simulink subsystem "PvtSubSys_VSM_LCKIE"  (R2020b)
settings: Solver=VariableStepAuto  StartTime=0.0  StopTime=10.0  RelTol=1e-3
values from neighbouring files (symbols this model uses):
  P_VSM_LCKIE_ClassInput = 0.0    [LCKIE.sldd]
  P_VSM_LCKIE_Laneoffset : value not decoded    [LCKIE.sldd]
  P_VSM_LCKIE_Laneoffset_BP : value not decoded    [LCKIE.sldd]
  P_VSM_LCKIE_LatC_DisOffofLanWidth : value not decoded    [LCKIE.sldd]
  P_VSM_LCKIE_LatC_DisOffofSpd : value not decoded    [LCKIE.sldd]
  P_VSM_LCKIE_LatC_DisSW = 0.0    [LCKIE.sldd]
  P_VSM_LCKIE_LatC_LanWidth : value not decoded    [LCKIE.sldd]
  P_VSM_LCKIE_LATC_LimitDis : value not decoded    [LCKIE.sldd]
  P_VSM_LCKIE_LATC_LimitDis_BP : value not decoded    [LCKIE.sldd]
  P_VSM_LCKIE_LatC_LimitDisEgoToObjSelt = 1.5    [LCKIE.sldd]
  P_VSM_LCKIE_LatC_LimitEgoToOppLane = 0.3    [LCKIE.sldd]
  P_VSM_LCKIE_LatC_maxLimitDisREToLane = 2.5    [LCKIE.sldd]
  P_VSM_LCKIE_LatC_minLimitDisREToLane = 1.2    [LCKIE.sldd]
  P_VSM_LCKIE_LatC_MoveEnableDis = 0.0    [LCKIE.sldd]
  P_VSM_LCKIE_LatC_RESafDis = 0.8    [LCKIE.sldd]
  P_VSM_LCKIE_LatC_SafeDisofLanWidth : value not decoded    [LCKIE.sldd]
  P_VSM_LCKIE_LatC_Spd : value not decoded    [LCKIE.sldd]
  P_VSM_LCKIE_LongC_d1 : value not decoded    [LCKIE.sldd]
  P_VSM_LCKIE_LongC_d2 : value not decoded    [LCKIE.sldd]
  P_VSM_LCKIE_LongC_DetaSpd : value not decoded    [LCKIE.sldd]
  P_VSM_LCKIE_LongC_DirecChangeDis = 20.0    [LCKIE.sldd]
  P_VSM_LCKIE_LongC_FleetOff = 80.0    [LCKIE.sldd]
  P_VSM_LCKIE_LongC_maxDis = 80.0    [LCKIE.sldd]
  P_VSM_LCKIE_LongC_minDis = 50.0    [LCKIE.sldd]
  P_VSM_LCKIE_LongC_ShutDownLongDis = -25.0    [LCKIE.sldd]
  P_VSM_LCKIE_LongC_ShutDownTTC = -4.0    [LCKIE.sldd]
  P_VSM_LCKIE_LongC_Spd : value not decoded    [LCKIE.sldd]
  P_VSM_LCKIE_LongC_toff = 10.0    [LCKIE.sldd]
  P_VSM_LCKIE_OFC_ActDis = 10.0    [LCKIE.sldd]
  P_VSM_LCKIE_OFC_DownDis = 10.0    [LCKIE.sldd]
  P_VSM_LCKIE_OFC_DownTTC = 5.0    [LCKIE.sldd]
  P_VSM_LCKIE_OFC_SafDis = 10.0    [LCKIE.sldd]
  P_VSM_LCKIE_OFC_Toff = 3.0    [LCKIE.sldd]
  P_VSM_LCKIE_ORC_LatDis = 1.8    [LCKIE.sldd]
  P_VSM_LCKIE_ORC_LimitDis1 = -30.0    [LCKIE.sldd]
  P_VSM_LCKIE_ORC_LimitDis2 = -10.0    [LCKIE.sldd]
  P_VSM_LCKIE_ORC_LimitTTC = 10.0    [LCKIE.sldd]
  P_VSM_LCKIE_ORC_LowSpd = -5.0    [LCKIE.sldd]
  P_VSM_LCKIE_POC_Delaytime : value not decoded    [LCKIE.sldd]
  P_VSM_LCKIE_POC_detaSpd : value not decoded    [LCKIE.sldd]
  P_VSM_LCKIE_POC_LimitDis = -15.0    [LCKIE.sldd]
  P_VSM_LCKIE_POC_LimitTTC = 2.0    [LCKIE.sldd]
  P_VSM_LCKIE_State_CurveMax = 0.005    [LCKIE.sldd]
  P_VSM_LCKIE_State_CurveMin = 0.0055555555555555558    [LCKIE.sldd]
  P_VSM_LCKIE_State_detaspd = 1.39    [LCKIE.sldd]
  P_VSM_LCKIE_State_detaspd_enable = 1.0    [LCKIE.sldd]
  P_VSM_LCKIE_State_DriverInputTrqValue_enable = 1.0    [LCKIE.sldd]
  P_VSM_LCKIE_State_ELKObjClc = 1.0    [LCKIE.sldd]
  P_VSM_LCKIE_State_HWASts_disable = 1.0    [LCKIE.sldd]
  P_VSM_LCKIE_State_IEObjClc = 1.0    [LCKIE.sldd]
  P_VSM_LCKIE_State_IFVReady = 1.0    [LCKIE.sldd]
  P_VSM_LCKIE_State_lamb_enable = 1.0    [LCKIE.sldd]
  P_VSM_LCKIE_State_Lanecurve_enable = 1.0    [LCKIE.sldd]
  P_VSM_LCKIE_State_LaneWidth_enable = 1.0    [LCKIE.sldd]
  P_VSM_LCKIE_State_Off2on = 3.0    [LCKIE.sldd]
  P_VSM_LCKIE_State_OppObjClc = 1.0    [LCKIE.sldd]
  P_VSM_LCKIE_STATE_ORCObjenable = 0.0    [LCKIE.sldd]
  P_VSM_LCKIE_State_Vehspeed_enable = 1.0    [LCKIE.sldd]
  P_VSM_LCKIE_State_wiper_enable = 1.0    [LCKIE.sldd]
  P_VSM_LCKIE_tcycle = 0.02    [LCKIE.sldd]
undefined symbols (not defined in the file or in its folder): P_Global_Vehicle_Length_m, P_Global_VehicleWidthMin_m, P_VSM_LSMC_SampleTime, STATE
libraries: simulink x62
(part 1 of 5)
settings Model: Creator=GW00133806  LastModifiedBy=GW00201118

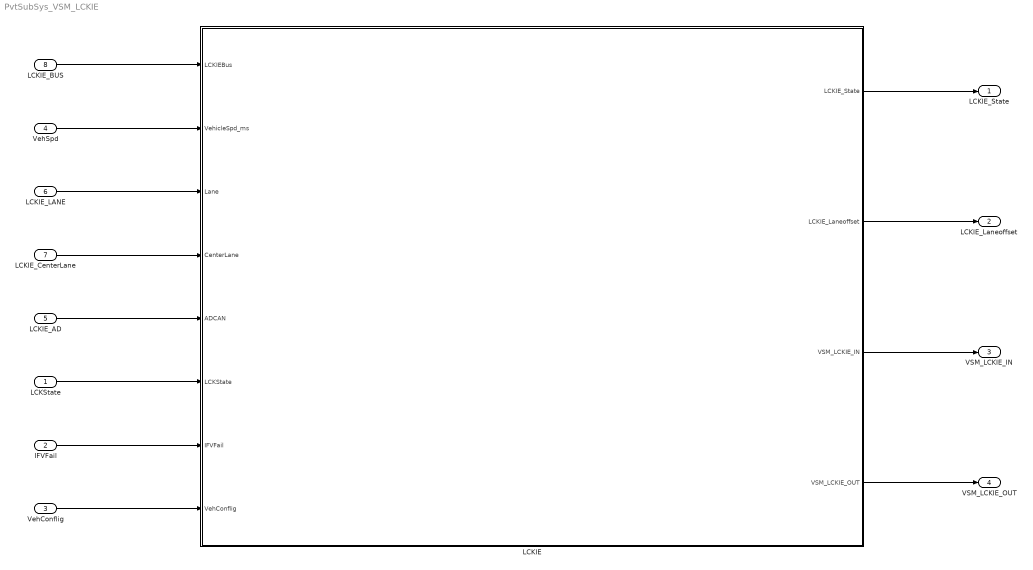
== system PvtSubSys_VSM_LCKIE ==
  LCKState : Inport
  IFVFail : Inport  Port=2
  VehConflig : Inport  Port=3
  VehSpd : Inport  Port=4
  LCKIE_AD : Inport  Port=5  OutDataTypeStr=Bus: LCKIE_AD  BusOutputAsStruct=on
  LCKIE_LANE : Inport  Port=6  BusOutputAsStruct=on
  LCKIE_CenterLane : Inport  Port=7  OutDataTypeStr=Bus: CenterLane  BusOutputAsStruct=on
  LCKIE_BUS : Inport  Port=8  OutDataTypeStr=Bus: TOS_LCKIE_BUS  BusOutputAsStruct=on
  LCKIE : Subsystem
  LCKIE_State : Outport
  LCKIE_Laneoffset : Outport  Port=2
  VSM_LCKIE_IN : Outport  Port=3
  VSM_LCKIE_OUT : Outport  Port=4
  wires:
  LCKIE/2(LCKIE_Laneoffset) -> LCKIE_Laneoffset/1
  LCKState/1 -> LCKIE/6(LCKState)
  LCKIE/3(VSM_LCKIE_IN) -> VSM_LCKIE_IN/1
  LCKIE_CenterLane/1 -> LCKIE/4(CenterLane)
  VehConflig/1 -> LCKIE/8(VehConflig)
  LCKIE/1(LCKIE_State) -> LCKIE_State/1
  LCKIE_BUS/1 -> LCKIE/1(LCKIEBus)
  VehSpd/1 -> LCKIE/2(VehicleSpd_ms)
  IFVFail/1 -> LCKIE/7(IFVFail)
  LCKIE/4(VSM_LCKIE_OUT) -> VSM_LCKIE_OUT/1
  LCKIE_LANE/1 -> LCKIE/3(Lane)
  LCKIE_AD/1 -> LCKIE/5(ADCAN)

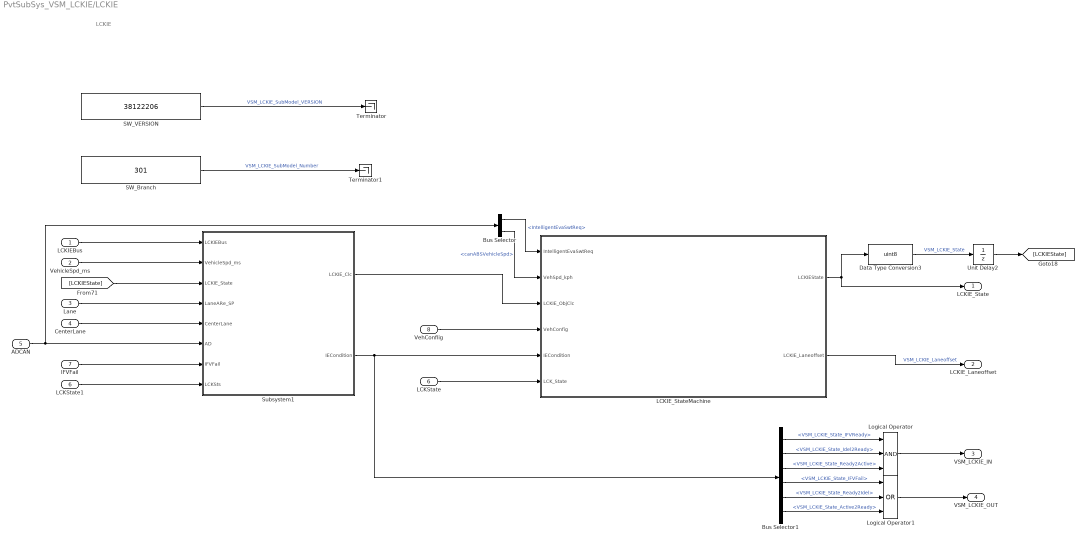
== system PvtSubSys_VSM_LCKIE/LCKIE ==
  note: LCKIE
  LCKIEBus : Inport
  VehicleSpd_ms : Inport  Port=2
  Lane : Inport  Port=3
  CenterLane : Inport  Port=4
  ADCAN : Inport  Port=5
  LCKState : Inport  Port=6
  IFVFail : Inport  Port=7
  VehConflig : Inport  Port=8
  Bus Selector : BusSelector  OutputSignals=IntelligentEvaSwtReq,canABSVehicleSpd
  Bus Selector1 : BusSelector  OutputSignals=VSM_LCKIE_State_IFVReady,VSM_LCKIE_State_Idel2Ready,VSM_LCKIE_State_Ready2Active,VSM_LCKIE_State_IFVFail,VSM_LCKIE_State_Ready2Idel,VSM_LCKIE_State_Active2Ready
  Data Type Conversion3 : DataTypeConversion  OutDataTypeStr=uint8
  LCKIE_StateMachine : Subsystem
  LCKState1 : InportShadow  Port=6
  Logical Operator : Logic  Inputs=3  AllPortsSameDT=off  OutDataTypeStr=boolean
  Logical Operator1 : Logic  Operator=OR  Inputs=3  AllPortsSameDT=off  OutDataTypeStr=boolean
  SW_Branch : Constant  Value=301  OutDataTypeStr=uint16
  SW_VERSION : Constant  Value=38122206  OutDataTypeStr=uint32
  Subsystem1 : Subsystem
  Terminator : Terminator
  Terminator1 : Terminator
  Unit Delay2 : UnitDelay  SampleTime=-1  HasFrameUpgradeWarning=on
  LCKIE_State : Outport
  LCKIE_Laneoffset : Outport  Port=2
  VSM_LCKIE_IN : Outport  Port=3
  VSM_LCKIE_OUT : Outport  Port=4
  wires:
  SW_Branch/1 -> Terminator1/1  "VSM_LCKIE_SubModel_Number"
  Bus Selector/1 -> LCKIE_StateMachine/1(IntelligentEvaSwtReq)  "<IntelligentEvaSwtReq>"
  Logical Operator1/1 -> VSM_LCKIE_OUT/1
  Logical Operator/1 -> VSM_LCKIE_IN/1
  Bus Selector1/6 -> Logical Operator1/3  "<VSM_LCKIE_State_Active2Ready>"
  Bus Selector1/5 -> Logical Operator1/2  "<VSM_LCKIE_State_Ready2Idel>"
  Bus Selector1/4 -> Logical Operator1/1  "<VSM_LCKIE_State_IFVFail>"
  Bus Selector1/3 -> Logical Operator/3  "<VSM_LCKIE_State_Ready2Active>"
  Bus Selector1/2 -> Logical Operator/2  "<VSM_LCKIE_State_Idel2Ready>"
  Bus Selector1/1 -> Logical Operator/1  "<VSM_LCKIE_State_IFVReady>"
  VehConflig/1 -> LCKIE_StateMachine/4(VehConfig)
  CenterLane/1 -> Subsystem1/5(CenterLane)
  Lane/1 -> Subsystem1/4(LaneARe_SP)
  VehicleSpd_ms/1 -> Subsystem1/2(VehicleSpd_ms)
  IFVFail/1 -> Subsystem1/7(IFVFail)
  Unit Delay2/1 -> [LCKIEState]
  ADCAN/1 -> Subsystem1/6(AD), Bus Selector/1
  LCKIE_StateMachine/1(LCKIEState) -> Data Type Conversion3/1, LCKIE_State/1
  Subsystem1/2(IECondition) -> Bus Selector1/1, LCKIE_StateMachine/5(IECondition)
  Subsystem1/1(LCKIE_Clc) -> LCKIE_StateMachine/3(LCKIE_ObjClc)
  Data Type Conversion3/1 -> Unit Delay2/1  "VSM_LCKIE_State"
  [LCKIEState] -> Subsystem1/3(LCKIE_State)
  LCKState/1 -> LCKIE_StateMachine/6(LCK_State)
  LCKIEBus/1 -> Subsystem1/1(LCKIEBus)
  LCKIE_StateMachine/2(LCKIE_Laneoffset) -> LCKIE_Laneoffset/1  "VSM_LCKIE_Laneoffset"
  SW_VERSION/1 -> Terminator/1  "VSM_LCKIE_SubModel_VERSION"
  LCKState1/1 -> Subsystem1/8(LCKSts)
  Bus Selector/2 -> LCKIE_StateMachine/2(VehSpd_kph)  "<canABSVehicleSpd>"

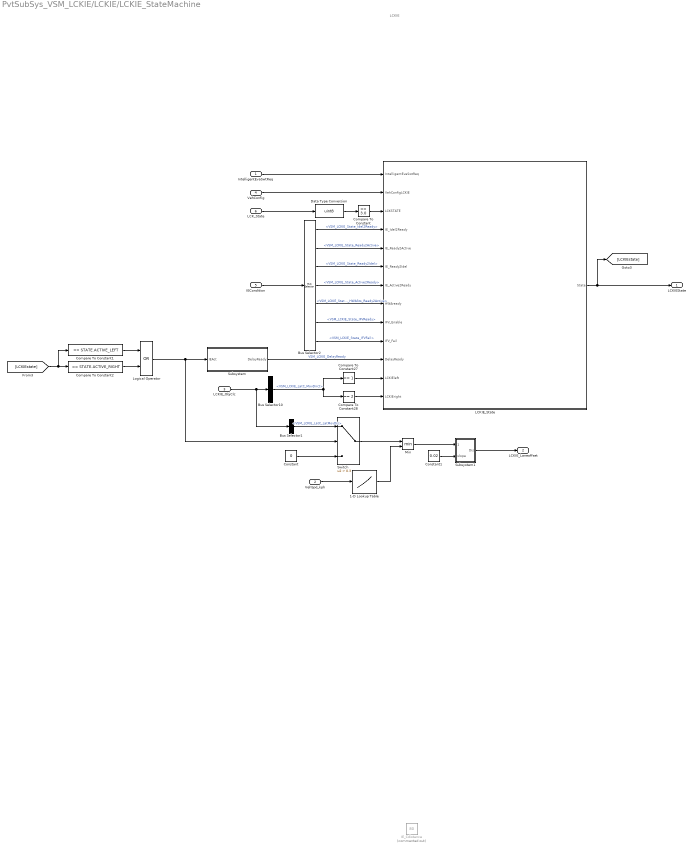
== system PvtSubSys_VSM_LCKIE/LCKIE/LCKIE_StateMachine ==
  note: LCKIE
  IntelligentEvaSwtReq : Inport
  VehSpd_kph : Inport  Port=2
  LCKIE_ObjClc : Inport  Port=3
  VehConfig : Inport  Port=4
  IECondition : Inport  Port=5
  LCK_State : Inport  Port=6
  1-D Lookup Table : Lookup_n-D  NumberOfTableDimensions=1  BreakpointsForDimension1=P_VSM_LCKIE_Laneoffset_BP  Table=P_VSM_LCKIE_Laneoffset  ExtrapMethod=Clip  UseLastTableValue=on  InternalRulePriority=Speed  RndMeth=Simplest  InputSameDT=on
  Bus Selector1 : BusSelector  OutputSignals=VSM_LCKIE_LatC_LatMovDis
  Bus Selector10 : BusSelector  OutputSignals=VSM_LCKIE_LatC_MovDirct
  Bus Selector2 : BusSelector  OutputSignals=VSM_LCKIE_State_Idel2Ready,VSM_LCKIE_State_Ready2Active,VSM_LCKIE_State_Ready2Idel,VSM_LCKIE_State_Active2Ready,VSM_LCKIE_State_HWASts_Ready2Active,VSM_LCKIE_State_IFVReady,VSM_LCKIE_State_IFVFail
  Compare To Constant : simulink/Logic and Bit Operations/Compare To Constant  relop===  const=3.0  OutDataTypeStr=boolean
  Compare To Constant1 : simulink/Logic and Bit Operations/Compare To Constant  relop===  const=STATE.ACTIVE_LEFT  OutDataTypeStr=boolean
  Compare To Constant2 : simulink/Logic and Bit Operations/Compare To Constant  relop===  const=STATE.ACTIVE_RIGHT  OutDataTypeStr=boolean
  Compare To Constant27 : simulink/Logic and Bit Operations/Compare To Constant  relop===  const=1  OutDataTypeStr=boolean
  Compare To Constant28 : simulink/Logic and Bit Operations/Compare To Constant  relop===  const=2  OutDataTypeStr=boolean
  Constant : Constant  Value=0
  Constant1 : Constant  Value=0.02  OutDataTypeStr=single
  Data Type Conversion : DataTypeConversion  OutDataTypeStr=uint8
  IE_Cdistance : Constant  Commented=on  Value=80
  LCKIE_State : Stateflow chart  TreatAsAtomicUnit=on
  Logical Operator : Logic  Operator=OR  AllPortsSameDT=off  OutDataTypeStr=boolean
  Min : MinMax  Inputs=2
  Subsystem : Subsystem
  Subsystem1 : Subsystem
  Switch : Switch  Criteria=u2 > Threshold  Threshold=0.3  OutDataTypeStr=single
  LCKIEState : Outport
  LCKIE_Laneoffset : Outport  Port=2
  wires:
  Compare To Constant/1 -> LCKIE_State/3(LCKSTATE)
  Switch/1 -> Min/1
  LCKIE_State/1(State) -> [LCKIEstate], LCKIEState/1
  Compare To Constant1/1 -> Logical Operator/1
  Compare To Constant2/1 -> Logical Operator/2
  Constant/1 -> Switch/3
  Compare To Constant28/1 -> LCKIE_State/13(LCKIEright)
  IntelligentEvaSwtReq/1 -> LCKIE_State/1(IntelligentEvaSwtReq)
  LCK_State/1 -> Data Type Conversion/1
  Compare To Constant27/1 -> LCKIE_State/12(LCKIEleft)
  Bus Selector10/1 -> Compare To Constant28/1, Compare To Constant27/1  "<VSM_LCKIE_LatC_MovDirct>"
  Data Type Conversion/1 -> Compare To Constant/1
  [LCKIEstate] -> Compare To Constant2/1, Compare To Constant1/1
  VehConfig/1 -> LCKIE_State/2(VehConfigLCKIE)
  Min/1 -> Subsystem1/1(DisLimmit)
  Bus Selector1/1 -> Switch/1  "<VSM_LCKIE_LatC_LatMovDis>"
  IECondition/1 -> Bus Selector2/1
  Bus Selector2/2 -> LCKIE_State/5(IE_Ready2Active)  "<VSM_LCKIE_State_Ready2Active>"
  Bus Selector2/1 -> LCKIE_State/4(IE_Idel2Ready)  "<VSM_LCKIE_State_Idel2Ready>"
  Bus Selector2/3 -> LCKIE_State/6(IE_Ready2Idel)  "<VSM_LCKIE_State_Ready2Idel>"
  Bus Selector2/4 -> LCKIE_State/7(IE_Active2Ready)  "<VSM_LCKIE_State_Active2Ready>"
  Bus Selector2/6 -> LCKIE_State/9(IFV_Enable)  "<VSM_LCKIE_State_IFVReady>"
  Bus Selector2/7 -> LCKIE_State/10(IFV_Fail)  "<VSM_LCKIE_State_IFVFail>"
  Subsystem1/1(Dis) -> LCKIE_Laneoffset/1
  Constant1/1 -> Subsystem1/2(slope)
  Bus Selector2/5 -> LCKIE_State/8(HWAready)  "<VSM_LCKIE_State_HWASts_Ready2Active>"
  Logical Operator/1 -> Switch/2, Subsystem/1(IEAct)
  Subsystem/1(DelayReady) -> LCKIE_State/11(DelayReady)  "VSM_LCKIE_DelayReady"
  LCKIE_ObjClc/1 -> Bus Selector1/1, Bus Selector10/1
  VehSpd_kph/1 -> 1-D Lookup Table/1
  1-D Lookup Table/1 -> Min/2

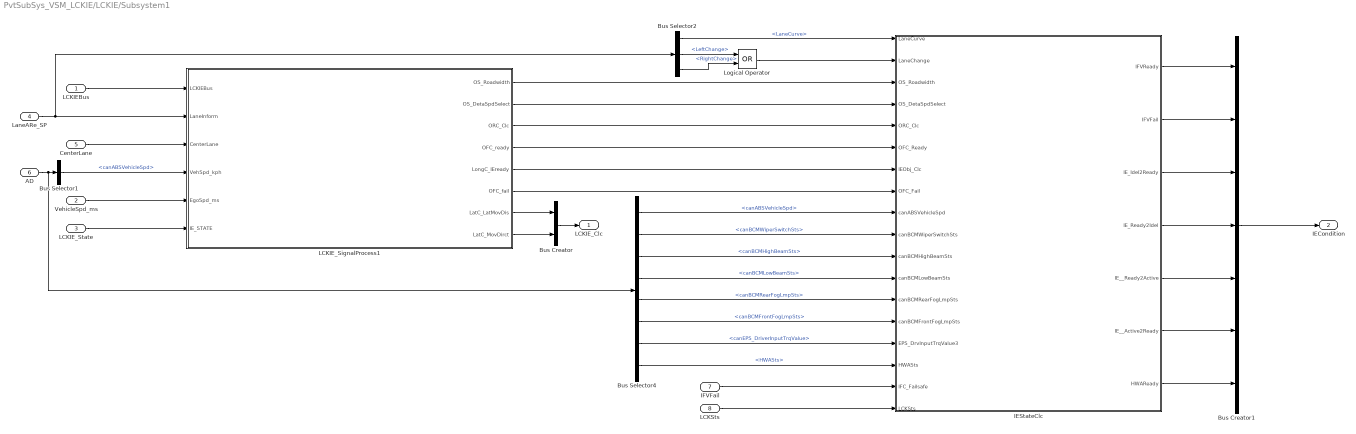
== system PvtSubSys_VSM_LCKIE/LCKIE/Subsystem1 ==
  LCKIEBus : Inport
  VehicleSpd_ms : Inport  Port=2
  LCKIE_State : Inport  Port=3
  LaneARe_SP : Inport  Port=4
  CenterLane : Inport  Port=5
  AD : Inport  Port=6
  IFVFail : Inport  Port=7
  LCKSts : Inport  Port=8
  Bus Creator : BusCreator  Inputs=2
  Bus Creator1 : BusCreator  Inputs=7
  Bus Selector1 : BusSelector  OutputSignals=canABSVehicleSpd
  Bus Selector2 : BusSelector  OutputSignals=LaneCurve,LeftChange,RightChange
  Bus Selector4 : BusSelector  OutputSignals=canABSVehicleSpd,canBCMWiperSwitchSts,canBCMHighBeamSts,canBCMLowBeamSts,canBCMRearFogLmpSts,canBCMFrontFogLmpSts,canEPS_DriverInputTrqValue,HWASts
  IEStateClc : Subsystem
  LCKIE_SignalProcess1 : Subsystem
  Logical Operator : Logic  Operator=OR  AllPortsSameDT=off  OutDataTypeStr=boolean
  LCKIE_Clc : Outport
  IECondition : Outport  Port=2
  wires:
  Logical Operator/1 -> IEStateClc/2(LaneChange)
  Bus Selector2/3 -> Logical Operator/2  "<RightChange>"
  LaneARe_SP/1 -> LCKIE_SignalProcess1/2(LaneInform), Bus Selector2/1
  LCKIE_SignalProcess1/5(LongC_IEready) -> IEStateClc/7(IEObj_Clc)
  LCKIE_SignalProcess1/4(OFC_ready) -> IEStateClc/6(OFC_Ready)
  LCKIE_SignalProcess1/3(ORC_Clc) -> IEStateClc/5(ORC_Clc)
  LCKIE_SignalProcess1/2(OS_DetaSpdSelect) -> IEStateClc/4(OS_DetaSpdSelect)
  LCKIE_SignalProcess1/6(OFC_fail) -> IEStateClc/8(OFC_Fail)
  LCKIE_SignalProcess1/1(OS_Roadwidth) -> IEStateClc/3(OS_Roadwidth)
  IEStateClc/1(IFVReady) -> Bus Creator1/1
  IEStateClc/6(IE__Active2Ready) -> Bus Creator1/6
  IEStateClc/2(IFVFail) -> Bus Creator1/2
  IEStateClc/5(IE__Ready2Active) -> Bus Creator1/5
  IEStateClc/3(IE_Idel2Ready) -> Bus Creator1/3
  IEStateClc/4(IE_Ready2Idel) -> Bus Creator1/4
  LCKIE_SignalProcess1/8(LatC_MovDirct) -> Bus Creator/2
  LCKIE_SignalProcess1/7(LatC_LatMovDis) -> Bus Creator/1
  VehicleSpd_ms/1 -> LCKIE_SignalProcess1/5(EgoSpd_ms)
  LCKIE_State/1 -> LCKIE_SignalProcess1/6(IE_STATE)
  CenterLane/1 -> LCKIE_SignalProcess1/3(CenterLane)
  LCKIEBus/1 -> LCKIE_SignalProcess1/1(LCKIEBus)
  Bus Selector1/1 -> LCKIE_SignalProcess1/4(VehSpd_kph)  "<canABSVehicleSpd>"
  Bus Creator/1 -> LCKIE_Clc/1
  IFVFail/1 -> IEStateClc/17(IFC_Failsafe)
  AD/1 -> Bus Selector1/1, Bus Selector4/1
  Bus Selector4/7 -> IEStateClc/15(EPS_DrvInputTrqValue3)  "<canEPS_DriverInputTrqValue>"
  Bus Selector4/6 -> IEStateClc/14(canBCMFrontFogLmpSts)  "<canBCMFrontFogLmpSts>"
  Bus Selector4/5 -> IEStateClc/13(canBCMRearFogLmpSts)  "<canBCMRearFogLmpSts>"
  Bus Selector4/4 -> IEStateClc/12(canBCMLowBeamSts)  "<canBCMLowBeamSts>"
  Bus Selector4/3 -> IEStateClc/11(canBCMHighBeamSts)  "<canBCMHighBeamSts>"
  Bus Selector4/2 -> IEStateClc/10(canBCMWiperSwitchSts)  "<canBCMWiperSwitchSts>"
  Bus Selector4/1 -> IEStateClc/9(canABSVehicleSpd)  "<canABSVehicleSpd>"
  Bus Creator1/1 -> IECondition/1
  Bus Selector2/1 -> IEStateClc/1(LaneCurve)  "<LaneCurve>"
  Bus Selector4/8 -> IEStateClc/16(HWASts)  "<HWASts>"
  IEStateClc/7(HWAReady) -> Bus Creator1/7
  Bus Selector2/2 -> Logical Operator/1  "<LeftChange>"
  LCKSts/1 -> IEStateClc/18(LCKSts)

== system PvtSubSys_VSM_LCKIE/LCKIE/LCKIE_StateMachine/Subsystem ==
  IEAct : Inport
  MATLAB Function : MATLAB Function  TreatAsAtomicUnit=on
  P_VSM_LCKIE_LatParaClc_Lane_max2midLaneWidth : Constant  Value=P_VSM_LCKIE_State_Off2on
  P_VSM_LCKIE_LatParaClc_Lane_max2midLaneWidth1 : Constant  Value=P_VSM_LCKIE_tcycle
  Unit Delay{,1..3} (4 alike) : UnitDelay  SampleTime=-1  HasFrameUpgradeWarning=on
  DelayReady : Outport
  wires:
  IEAct/1 -> Unit Delay3/1
  Unit Delay/1 -> MATLAB Function/2(IEActK1)
  MATLAB Function/2(flg) -> Unit Delay2/1
  P_VSM_LCKIE_LatParaClc_Lane_max2midLaneWidth1/1 -> MATLAB Function/3(tcycle)
  P_VSM_LCKIE_LatParaClc_Lane_max2midLaneWidth/1 -> MATLAB Function/4(t_offset)
  Unit Delay1/1 -> MATLAB Function/6(delaytimeK1)
  MATLAB Function/3(delaytime) -> Unit Delay1/1
  Unit Delay2/1 -> MATLAB Function/5(flgK1)
  MATLAB Function/1(DelayReady) -> DelayReady/1
  Unit Delay3/1 -> Unit Delay/1, MATLAB Function/1(IEAct)

== system PvtSubSys_VSM_LCKIE/LCKIE/LCKIE_StateMachine/Subsystem1 ==
  DisLimmit : Inport
  slope : Inport  Port=2
  MATLAB Function : MATLAB Function  TreatAsAtomicUnit=on
  Unit Delay : UnitDelay  SampleTime=-1  HasFrameUpgradeWarning=on
  Dis : Outport
  wires:
  Unit Delay/1 -> MATLAB Function/3(DisK1)
  DisLimmit/1 -> MATLAB Function/1(DisLimmit)
  slope/1 -> MATLAB Function/2(slope)
  MATLAB Function/1(Dis) -> Dis/1, Unit Delay/1
